simulink model "GlbDa_TrqDem"  (R2016b)
settings: configuration reference "CodeGenConfigSet" (kept outside this file)
values from neighbouring files (symbols this model uses):
  GlbDa_stTrqDem_C = Calibration.Parameter    [init_GlbDa_TrqDem.m]    (also in init_GlbDa_TrqDem_SIL.m = Simulink.Parameter)
libraries: simulink x6
settings Model: Creator=Wollf  LastModifiedBy=lenovo
settings ConfigSetRef: SourceLocation=Base Workspace

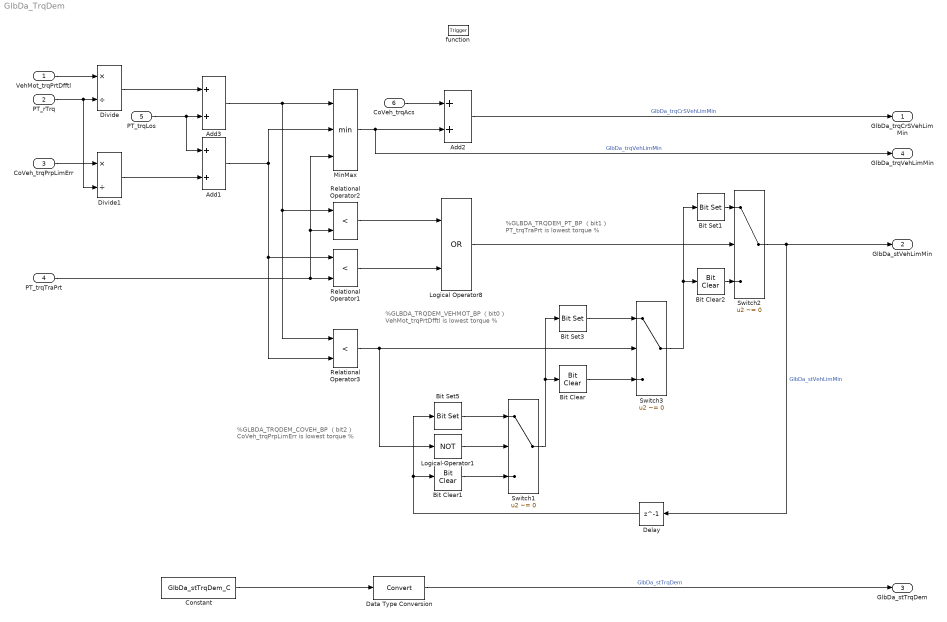
== system GlbDa_TrqDem ==
  note: %GLBDA_TRQDEM_VEHMOT_BP （bit0）
      | VehMot_trqPrtDfftl is lowest torque %
  note: %GLBDA_TRQDEM_COVEH_BP （bit2）
      | CoVeh_trqPrpLimErr is lowest torque %
  note: %GLBDA_TRQDEM_PT_BP （bit1）
      | PT_trqTraPrt is lowest torque %
  VehMot_trqPrtDfftl : Inport  Tag=Nm  Description=Differential protection torque  OutMin=-3000  OutMax=3000  OutDataTypeStr=Trq_Nm
  PT_rTrq : Inport  Description=Powertrain torque ratio  Port=2  OutMin=-100  OutMax=100  OutDataTypeStr=TransRatio
  CoVeh_trqPrpLimErr : Inport  Tag=Nm  Description=limitation torque for propulsion at system error  Port=3  OutMin=-3000  OutMax=3000  OutDataTypeStr=Trq_Nm
  PT_trqTraPrt : Inport  Tag=Nm  Description=Maximum allowed inner torque  Port=4  OutMin=-3000  OutMax=3000  OutDataTypeStr=Trq_Nm
  PT_trqLos : Inport  Tag=Nm  Description=Parameter for loss torque of the drive train  Port=5  OutMin=-3000  OutMax=3000  OutDataTypeStr=Trq_Nm
  CoVeh_trqAcs : Inport  Tag=Nm  Description=message for demand of accessories  Port=6  OutMin=-3276.8  OutMax=3276.7  OutDataTypeStr=Trq_Nm
  function : TriggerPort  TriggerType=function-call  VariantControl=Variant
  Add1 : Sum  SaturateOnIntegerOverflow=on  InputSameDT=on
  Add2 : Sum  SaturateOnIntegerOverflow=on  InputSameDT=on
  Add3 : Sum  SaturateOnIntegerOverflow=on  InputSameDT=on
  Bit Clear : simulink/Logic and Bit Operations/Bit Clear  iBit=0
  Bit Clear1 : simulink/Logic and Bit Operations/Bit Clear  iBit=2
  Bit Clear2 : simulink/Logic and Bit Operations/Bit Clear  iBit=1
  Bit Set1 : simulink/Logic and Bit Operations/Bit Set  iBit=1
  Bit Set3 : simulink/Logic and Bit Operations/Bit Set  iBit=0
  Bit Set5 : simulink/Logic and Bit Operations/Bit Set  iBit=2
  Constant : Constant  Value=GlbDa_stTrqDem_C
  Data Type Conversion : DataTypeConversion
  Delay : Delay  DelayLength=1  InitialCondition=0
  Divide : Product  Inputs=*/  OutDataTypeStr=Inherit: Inherit via back propagation  SaturateOnIntegerOverflow=on
  Divide1 : Product  Inputs=*/  OutDataTypeStr=Inherit: Inherit via back propagation  SaturateOnIntegerOverflow=on
  Logical Operator1 : Logic  Operator=NOT  OutDataTypeStr=boolean
  Logical Operator8 : Logic  Operator=OR  OutDataTypeStr=boolean
  MinMax : MinMax  Inputs=3  SaturateOnIntegerOverflow=on  InputSameDT=on
  Relational Operator1 : RelationalOperator  Operator=<  OutDataTypeStr=boolean  RndMeth=Simplest  InputSameDT=on
  Relational Operator2 : RelationalOperator  Operator=<  OutDataTypeStr=boolean  RndMeth=Simplest  InputSameDT=on
  Relational Operator3 : RelationalOperator  Operator=<  OutDataTypeStr=boolean  RndMeth=Simplest  InputSameDT=on
  Switch1 : Switch  Criteria=u2 ~= 0  SaturateOnIntegerOverflow=on  InputSameDT=on
  Switch2 : Switch  Criteria=u2 ~= 0  SaturateOnIntegerOverflow=on  InputSameDT=on
  Switch3 : Switch  Criteria=u2 ~= 0  SaturateOnIntegerOverflow=on  InputSameDT=on
  GlbDa_trqCrSVehLimMin : Outport  Tag=Nm  Description=current limitation torque from GlbDa on torque level crankshaft  OutMin=-3276.8  OutMax=3276.7  OutDataTypeStr=Trq_Nm
  GlbDa_stVehLimMin : Outport  Description=Current limitation state from GlbDa  Port=2  OutMin=0  OutMax=255  OutDataTypeStr=State_uint8
  GlbDa_stTrqDem : Outport  Description=contains highest prior function with torque demand  Port=3  OutMin=0  OutMax=4294967295  OutDataTypeStr=State_uint32
  GlbDa_trqVehLimMin : Outport  Tag=Nm  Description=Offset for Internal and External Speed Limitation  Port=4  OutMin=-3276.8  OutMax=3276.7  OutDataTypeStr=Trq_Nm
  wires:
  Logical Operator8/1 -> Switch2/2
  Switch2/1 -> GlbDa_stVehLimMin/1, Delay/1  "GlbDa_stVehLimMin"
  VehMot_trqPrtDfftl/1 -> Divide/1
  PT_rTrq/1 -> Divide1/2, Divide/2
  CoVeh_trqPrpLimErr/1 -> Divide1/1
  Divide/1 -> Add3/1
  Bit Clear/1 -> Switch3/3
  Bit Set3/1 -> Switch3/1
  Add2/1 -> GlbDa_trqCrSVehLimMin/1  "GlbDa_trqCrSVehLimMin"
  Switch3/1 -> Bit Clear2/1, Bit Set1/1
  CoVeh_trqAcs/1 -> Add2/1
  PT_trqLos/1 -> Add1/1, Add3/2
  MinMax/1 -> GlbDa_trqVehLimMin/1, Add2/2  "GlbDa_trqVehLimMin"
  Divide1/1 -> Add1/2
  Relational Operator1/1 -> Logical Operator8/2
  Add3/1 -> MinMax/1, Relational Operator3/1, Relational Operator2/1
  Add1/1 -> Relational Operator3/2, Relational Operator1/1, MinMax/2
  PT_trqTraPrt/1 -> MinMax/3, Relational Operator2/2, Relational Operator1/2
  Relational Operator2/1 -> Logical Operator8/1
  Bit Set1/1 -> Switch2/1
  Bit Clear1/1 -> Switch1/3
  Bit Set5/1 -> Switch1/1
  Relational Operator3/1 -> Logical Operator1/1, Switch3/2
  Switch1/1 -> Bit Clear/1, Bit Set3/1
  Logical Operator1/1 -> Switch1/2
  Bit Clear2/1 -> Switch2/3
  Delay/1 -> Bit Clear1/1, Bit Set5/1
  Constant/1 -> Data Type Conversion/1
  Data Type Conversion/1 -> GlbDa_stTrqDem/1  "GlbDa_stTrqDem"
